simulink model "Optical_Flow_Test"  (Simulink 10.0)
settings: Solver=VariableStepAuto  StartTime=0.0  StopTime=10  RelTol=1e-3
model workspace (MAT data in the model file):
  BBox_Area1 : num (value not decoded)
undefined symbols (not defined in the file): Horn, magnitude, none, Rec, Schunck, SDTV, strel, videoinput
libraries: imaqlib x2, visionanalysis x2, dspstat3 x2, visionconversions x1, dspsigattribs x1, visionstatistics x1, simulink x1, dspmtrx3 x1, dspindex x1, visiontextngfix x1, visionsinks x1, visionmorphops x1
settings Model: Creator=danie  LastModifiedBy=danie
settings DataIOCC: SaveFormat=Dataset  ReturnWorkspaceOutputs=on
settings OptimizationCC: LifeSpan=auto
settings DebuggingCC: UnderspecifiedInitializationDetection=Simplified  MergeDetectMultiDrivingBlocksExec=error  SFUnexpectedBacktrackingDiag=error  SFNoUnconditionalDefaultTransitionDiag=error  SFExecutionAtInitializationDiag=warning  ArithmeticOperatorsInVariantConditions=error
settings HardwareCC: ProdBitPerPointer=64  ProdBitPerSizeT=64  ProdBitPerPtrDiffT=64  ProdLargestAtomicFloat=Float  ProdIntDivRoundTo=Zero  ProdEndianess=LittleEndian  ProdWordSize=64  ProdHWDeviceType=Intel->x86-64 (Windows64)
settings ModelReferenceCC: PropagateSignalLabelsOutOfModel=on
settings SFSimCC: SimUseLocalCustomCode=on  CustomCodeUndefinedFunction=FilterOut
settings RTWCC: RTWUseLocalCustomCode=on
settings CodeAppCC: StateflowObjectComments=off
settings GRTTargetCC: TargetLangStandard=C99 (ISO)  CombineOutputUpdateFcns=on  GRTInterface=off
settings ConfigComp: CovMetricSettings=dwe  CovHtmlReporting=off  CovSaveCumulativeToWorkspaceVar=off  CovSaveSingleToWorkspaceVar=off

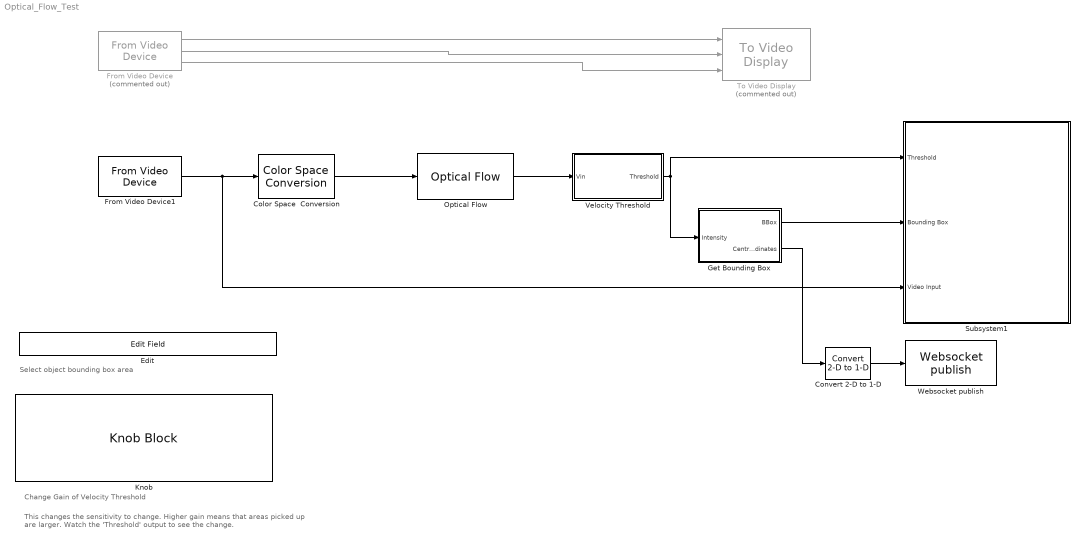
== system Optical_Flow_Test ==
  note: This changes the sensitivity to change. Higher gain means that areas picked
      | up are larger. Watch the 'Threshold' output to see the change.
  note: Change Gain of Velocity Threshold
  note: Select object bounding box area
  Color Space  Conversion : visionconversions/Color Space  Conversion  conversion=Obsolete  conversionActive=R'G'B' to intensity  wp_str=D65  rec=Rec. 601 (SDTV)  sys=1125/60/2:1  imagePorts=One multidimensional signal
  Convert 2-D to 1-D : dspsigattribs/Convert 2-D to 1-D
      settings: SourceProductName=DSP System Toolbox  SourceProductBaseCode=DS
  Edit : EditField  LabelPosition=Bottom  ShowInitialText=on  Alignment=Center
  From Video Device : imaqlib/From Video Device  Commented=on  DeviceMenu=winvideo 1 (USB_Camera)  Device=winvideo 1 (USB_Camera)  ObjConstructor=videoinput('winvideo', 1)  VideoFormatMenu=MJPG_1920x1080  VideoFormat=MJPG_1920x1080  VideoSource=input1  ROIPosition=[0 0 1080 1920]  EnableHWTrigger=off  TriggerConfiguration=none/none  SampleTime=1/30  OutputPortsMode=Separate color signals  DataType=double  CanDoHWTrigger=no  ReturnedColorSpace=rgb  BlockHandle=4.0002  ROIWidth=1920  ROIHeight=1080  ROIColumn=0  ROIRow=0  EngXMLPath=E:\Matlab\toolbox\imaq\imaq\private  DevXMLPath=C:\ProgramData\MATLAB\SupportPackages\R2019b\toolbox\imaq\supportpackages\genericvideo\adaptor\win64  EngLibPath=E:\Matlab\toolbox\imaq\imaqblks\imaqmex\win64  ColorSpace=rgb  BayerSensorAlignment=grbg  ImaqMode=off
      settings: SourceProductName=Image Acquisition Toolbox
  From Video Device1 : imaqlib/From Video Device  DeviceMenu=winvideo 1 (USB_Camera)  Device=winvideo 1 (USB_Camera)  ObjConstructor=videoinput('winvideo', 1)  VideoFormatMenu=MJPG_1920x1080  VideoFormat=MJPG_1920x1080  VideoSource=input1  ROIPosition=[0 0 1080 1920]  EnableHWTrigger=off  TriggerConfiguration=none/none  SampleTime=1/30  OutputPortsMode=One multidimensional signal  DataType=single  CanDoHWTrigger=no  ReturnedColorSpace=rgb  BlockHandle=4.0002  ROIWidth=1920  ROIHeight=1080  ROIColumn=0  ROIRow=0  EngXMLPath=E:\Matlab\toolbox\imaq\imaq\private  DevXMLPath=C:\ProgramData\MATLAB\SupportPackages\R2019b\toolbox\imaq\supportpackages\genericvideo\adaptor\win64  EngLibPath=E:\Matlab\toolbox\imaq\imaqblks\imaqmex\win64  ColorSpace=rgb  BayerSensorAlignment=grbg  ImaqMode=off
      settings: SourceProductName=Image Acquisition Toolbox
  Get Bounding Box : Subsystem
  Knob : KnobBlock  ScaleMin=1  ScaleMax=10
  Optical Flow : visionanalysis/Optical Flow  method=Horn-Schunck  gradMethod=Difference filter [-1 1]  which2img=Current frame and N-th frame back  N=1  lambda=1  numInports=3  sigmaS=1.5  sigmaW=1  discardNormalFlow=off  outputCurrentImage=off  stop_criteria=When maximum number of iterations is reached  maxIter=10  maxAllowAbsDiff=eps  outVelForm=Horizontal and vertical components in complex form  eigTh=0.0039  roundingMode=Nearest  overflowMode=on  prodOutputMode=Binary point scaling  prodOutputWordLength=32  prodOutputFracLength=20  prodOutputSlope=2^-20  accumSlope=2^-20  memorySlope=2^-20  firstCoeffSlope=2^-20  outputMode=Binary point scaling  outputWordLength=32  outputFracLength=20  outputSlope=2^-20
      settings: SourceProductName=Computer Vision Toolbox  SourceProductBaseCode=VP
  Subsystem1 : Subsystem
  To Video Display : visionsinks/To Video Display  Commented=on  windowSizeMode=Normal  openAtMdlStart=on  fullScreen=off  videoWindowX=536805376  videoWindowY=536805376  saveWindowSize=off  videoWindowWidth=2147483647  videoWindowHeight=2147483647  inputColorFormat=RGB  inputType=Obsolete  imagePorts=Separate color signals  OutputDevice=On-screen video monitor  dataOrg=Column-major  isWindowOpen=off
      settings: SourceProductName=Computer Vision Toolbox
  Velocity Threshold : Subsystem
  Websocket publish : raspberrypilib/Websocket publish  UniqueBlockID=webPub 1  IPAddress=127.0.0.1  Port=9000  NumberOfSignals=1
      settings: SourceProductName=Simulink Support Package for Raspberry Pi Hardware  SourceProductBaseCode=RASPPI
  wires:
  From Video Device/1 -> To Video Display/1
  From Video Device/2 -> To Video Display/2
  From Video Device/3 -> To Video Display/3
  From Video Device1/1 -> Subsystem1/3(Video Input), Color Space  Conversion/1
  Color Space  Conversion/1 -> Optical Flow/1
  Velocity Threshold/1(Threshold) -> Get Bounding Box/1(Intensity), Subsystem1/1(Threshold)
  Optical Flow/1 -> Velocity Threshold/1(Vin)
  Get Bounding Box/1(BBox) -> Subsystem1/2(Bounding Box)
  Convert 2-D to 1-D/1 -> Websocket publish/1
  Get Bounding Box/2(Central Coordinates) -> Convert 2-D to 1-D/1

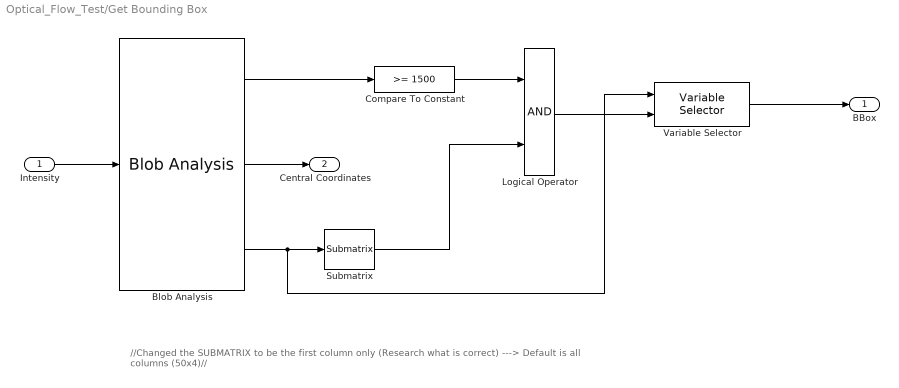
== system Optical_Flow_Test/Get Bounding Box ==
  note: //Changed the SUBMATRIX to be the first column only (Research what is correct) ---> Default is all columns (50x4)//
  Intensity : Inport
  Blob Analysis : visionstatistics/Blob Analysis  Tag=vipblks_row_conv  area=on  centroid=on  bBox=on  majorAxis=off  minorAxis=off  angle=off  eccentricity=off  equivDiameterSq=off  extent=off  perimeter=off  outDT=double  conn=8  isLabel=off  maxBlobs=50  warnIfNumBlobsExceeded=on  isCount=off  useMinArea=off  minArea=0  useMaxArea=off  maxArea=intmax('uint32')  excludeBorderBlob=off  isOutVarDim=off  isFill=on  fillValues=-1  roundingMode=Floor  overflowMode=off  prodOutputMode=Binary point scaling  prodOutputWordLength=32  prodOutputFracLength=16  prodOutputSlope=2^-16  accumMode=Binary point scaling  accumWordLength=32  accumFracLength=0  accumSlope=2^0  outputMode=Binary point scaling  outputWordLength=32  outputFracLength=16  outputSlope=2^-16  memorySlope=2^-16  firstCoeffMode=Binary point scaling  firstCoeffWordLength=16  firstCoeffFracLength=14  firstCoeffSlope=2^-14  secondCoeffMode=Binary point scaling  secondCoeffWordLength=32  secondCoeffFracLength=16  secondCoeffSlope=2^-16
      settings: SourceProductName=Computer Vision Toolbox
  Compare To Constant : simulink/Logic and Bit Operations/Compare To Constant  relop=>=  const=1500  OutDataTypeStr=boolean
  Logical Operator : Logic  AllPortsSameDT=off  OutDataTypeStr=boolean
  Submatrix : dspmtrx3/Submatrix  RowSpan=All rows  RowStartMode=First  RowStartIndex=1  RowEndMode=Last  RowEndIndex=1  ColSpan=One column  ColStartMode=First  ColStartIndex=1  ColEndMode=Last  ColEndIndex=1
  Variable Selector : dspindex/Variable Selector  NumInputs=1  rowsOrCols=Rows  IdxMode=Variable  Elements=[1 3]  ZerOneIdxMode=One-based  errmode=Clip Index  FillMode=on  FillValues=0
  BBox : Outport
  Central Coordinates : Outport  Port=2
  wires:
  Intensity/1 -> Blob Analysis/1
  Blob Analysis/3 -> Variable Selector/1, Submatrix/1
  Compare To Constant/1 -> Logical Operator/1
  Submatrix/1 -> Logical Operator/2
  Logical Operator/1 -> Variable Selector/2
  Variable Selector/1 -> BBox/1
  Blob Analysis/2 -> Central Coordinates/1
  Blob Analysis/1 -> Compare To Constant/1

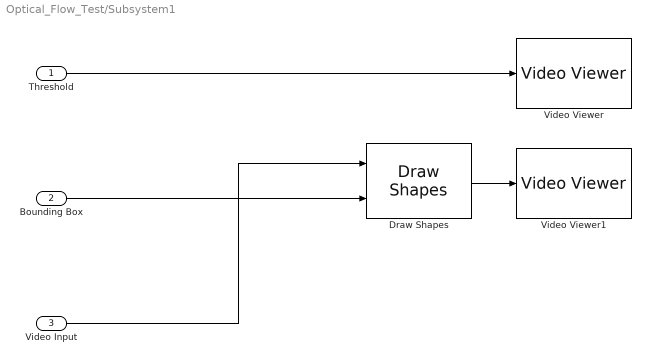
== system Optical_Flow_Test/Subsystem1 ==
  Threshold : Inport
  Bounding Box : Inport  Port=2
  Video Input : Inport  Port=3
  Draw Shapes : visiontextngfix/Draw Shapes  shape=Rectangles  fill=off  lineWidth=1  fillClrSource=Specify via dialog  display=User-specified value  intensity=200  color=[0 255 0]  opacity=0.6  viewport=Entire image  antialiasing=off  inType=Obsolete  imagePorts=One multidimensional signal  roundingMode=Floor  overflowMode=off  memoryMode=Specify word length  memoryWordLength=16  prodOutputMode=Binary point scaling  prodOutputWordLength=32  prodOutputFracLength=14  prodOutputSlope=2^-14  accumSlope=2^-14  memoryFracLength=15
      settings: SourceProductName=Computer Vision Toolbox
  Video Viewer : VideoViewer  FigPos=[962 1037 958 409]
  Video Viewer1 : VideoViewer  FigPos=[4 528 958 409]
  wires:
  Threshold/1 -> Video Viewer/1
  Draw Shapes/1 -> Video Viewer1/1
  Video Input/1 -> Draw Shapes/1
  Bounding Box/1 -> Draw Shapes/2

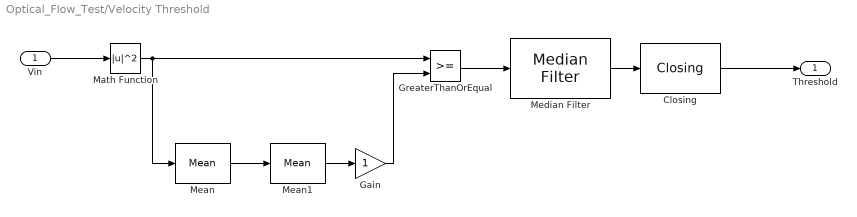
== system Optical_Flow_Test/Velocity Threshold ==
  Vin : Inport
  Closing : visionmorphops/Closing  nhoodsrc=Specify via dialog  strel=strel('line',5,45)
      settings: SourceProductName=Computer Vision Toolbox  SourceProductBaseCode=VP
  Gain : Gain
  GreaterThanOrEqual : RelationalOperator  OutDataTypeStr=boolean  RndMeth=Simplest
  Math Function : Math  Operator=magnitude^2  SignedPower=off  SaturateOnIntegerOverflow=on
  Mean : dspstat3/Mean  run=off  InputProcessing=Columns as channels (frame based)  reset_popup=None  directionMode=Entire input  dimension=1  roiEnable=off  roiType=Rectangles  roiPortion=Entire ROI  roiOutput=Individual statistics for each ROI  roiFlag=off  roundingMode=Floor  overflowMode=off  outputDataTypeStr=Inherit: Same as accumulator  outputMin=[]  outputMax=[]  outputLastDataTypeStr=Inherit: Same as accumulator
  Mean1 : dspstat3/Mean  run=on  InputProcessing=Columns as channels (frame based)  reset_popup=None  directionMode=Each column  dimension=1  roiEnable=off  roiType=Rectangles  roiPortion=Entire ROI  roiOutput=Individual statistics for each ROI  roiFlag=off  roundingMode=Floor  overflowMode=off  outputDataTypeStr=Inherit: Same as accumulator  outputMin=[]  outputMax=[]  outputLastDataTypeStr=Inherit: Same as accumulator
  Median Filter : visionanalysis/Median Filter  nghbood=[3 3]  outSize=Same as input port I  padType=Constant  padSrc=Specify via dialog  padVal=0  roundingMode=Floor  overflowMode=off  prodOutputSlope=2^-30  accumSlope=2^-30  outputSlope=2^-15
      settings: SourceProductName=Computer Vision Toolbox  SourceProductBaseCode=VP
  Threshold : Outport
  wires:
  Vin/1 -> Math Function/1
  Math Function/1 -> Mean/1, GreaterThanOrEqual/1
  Mean/1 -> Mean1/1
  Mean1/1 -> Gain/1
  Gain/1 -> GreaterThanOrEqual/2
  GreaterThanOrEqual/1 -> Median Filter/1
  Median Filter/1 -> Closing/1
  Closing/1 -> Threshold/1
